simulink library "Lib_EMTAT"  (R2021b)
settings: Solver=VariableStepAuto  StartTime=0.0  StopTime=10.0  RelTol=1e-3
undefined symbols (not defined in the file or in its folder): A_M, B_M, Cj, component_degradation_input, Cs, E0_M, f_sw, K_M, MWS, Q_M, Q_rr, r_c, r_D, R_M, Rj, Ru, SNR_DX_M, SNR_IC_M, SNR_Mn_M, SNR_Mx_M, SOC_Init_M, u_ce0, u_D0
libraries: $bdroot x82, simulink x23, Lib_Dyn_StateSpace_EMTAT x3, PB_Library_Master_Working x1
(part 5 of 7)

== system Lib_EMTAT/Components/Power Flow/Mechanical Shaft ==
  note: Units
      | J : lb-ft-s^2
      | B : lb-ft-s
  T : Inport
  Fail? : Inport  Port=2
  N : Inport  Port=3
  Abs : Abs
  Bus Creator : BusCreator  Inputs=5
  Divide : Product  Inputs=*/
  Failure Determination : Subsystem
  Inertia (slug-ft^2 or lbf-ft-s^2) : Constant  Value=J
  RPM to rad/s : Gain  Gain=(2*pi)/60
  Shaft Break Failure : Subsystem
  Sum : Sum  Inputs=|+-
  "Viscous Damping Coefficient, lbf-ft-s" : Gain  Gain=B
  lbf-ft to Btu : Gain  Gain=0.00128507
  rad/s^2 to RPM/s : Gain  Gain=60/(2*pi)
  Outputs : Outport
  Heat : Outport  Port=2
  Ndot : Outport  Port=3
  wires:
  Shaft Break Failure/1("T ") -> Sum/1
  [SBFail] -> Bus Creator/5  "SBFail"
  RPM to rad/s/1 -> "Viscous Damping Coefficient, lbf-ft-s"/1
  [SBFail] -> Shaft Break Failure/1(Failed?)
  Fail?/1 -> Failure Determination/1(Fail?)
  Failure Determination/1(SBFail) -> [SBFail]
  N/1 -> RPM to rad/s/1, [N]
  [Ndot] -> Bus Creator/3  "Ndot"
  Inertia (slug-ft^2 or lbf-ft-s^2)/1 -> Divide/2
  Bus Creator/1 -> Outputs/1
  rad/s^2 to RPM/s/1 -> [Ndot], Ndot/1
  Divide/1 -> rad/s^2 to RPM/s/1
  [Tnet] -> Bus Creator/1  "Tnet"
  [N] -> Bus Creator/2  "N"
  [Heat] -> Bus Creator/4  "Heat"
  Abs/1 -> Heat/1, [Heat]
  Sum/1 -> [Tnet], Divide/1
  "Viscous Damping Coefficient, lbf-ft-s"/1 -> Sum/2, lbf-ft to Btu/1
  lbf-ft to Btu/1 -> Abs/1
  T/1 -> Shaft Break Failure/2(T)

== system Lib_EMTAT/Components/Power Flow/Power Supply (Set Voltage) ==
  V* : Inport
  Idmd : Inport  Port=2
  Bus Creator : BusCreator  Inputs=3
  Divide : Product  Inputs=**
  MATLAB Function : MATLAB Function  TreatAsAtomicUnit=on
  Outputs : Outport
  Vout : Outport  Port=2
  wires:
  [Pdmd] -> Bus Creator/3  "Pdmd"
  [Idmdsum] -> Bus Creator/2  "Idmdsum"
  [Vout] -> Bus Creator/1  "Vout"
  Divide/1 -> [Pdmd]
  Bus Creator/1 -> Outputs/1
  V*/1 -> Vout/1, Divide/1, [Vout]
  MATLAB Function/1(y) -> [Idmdsum], Divide/2  "Idmdsum"
  Idmd/1 -> MATLAB Function/1(u)

== system Lib_EMTAT/Components/Power Flow/Resistive Load Bank ==
  V : Inport
  "P* " : Inport  Port=2
  Fail? : Inport  Port=3
  Abs1 : Abs
  Bus Creator : BusCreator  Inputs=5
  Divide2 : Product  Inputs=**
  Failure Determination : Subsystem
  Fix Divide By Zero. : Subsystem
  Fix Divide By Zero.1 : Subsystem
  Open Circuit Failure - Line to Neutral Voltage : Subsystem
  Square : Math  Operator=square  SaturateOnIntegerOverflow=on
  Outputs : Outport
  Ploss : Outport  Port=2
  Iin : Outport  Port=3
  wires:
  Fix Divide By Zero.1/1(I) -> Open Circuit Failure - Line to Neutral Voltage/2(I)
  [OCFail] -> Open Circuit Failure - Line to Neutral Voltage/1(Failed?)
  Fail?/1 -> Failure Determination/1(Fail?)
  Failure Determination/1(OCFail) -> [OCFail]
  Abs1/1 -> Fix Divide By Zero./2(abs(Pset))
  Fix Divide By Zero./1(R) -> [R], Divide2/2
  Bus Creator/1 -> Outputs/1
  Square/1 -> Divide2/1, Fix Divide By Zero./1(I^2)
  "P* "/1 -> [Pset], Abs1/1, Fix Divide By Zero.1/2(Pset)  "Pset"
  V/1 -> [V], Fix Divide By Zero.1/1(V)  "V"
  Divide2/1 -> [Ploss], Ploss/1
  [V] -> Bus Creator/1  "V"
  [I] -> Bus Creator/2  "I"
  [Pset] -> Bus Creator/3  "Pset"
  [R] -> Bus Creator/4  "R"
  [Ploss] -> Bus Creator/5  "Ploss"
  Open Circuit Failure - Line to Neutral Voltage/1("I ") -> Square/1, [I], Iin/1

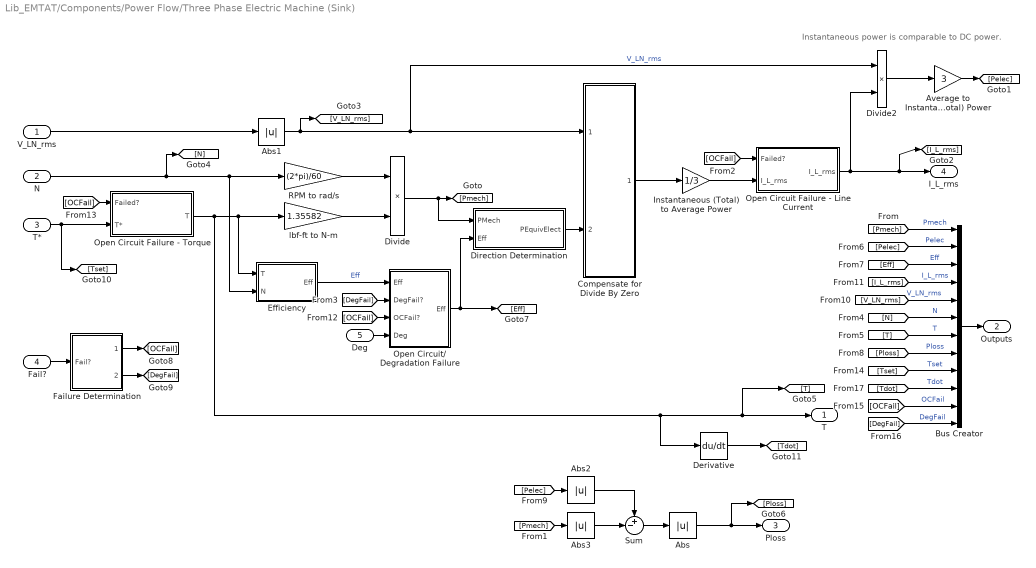
== system Lib_EMTAT/Components/Power Flow/Three Phase Electric Machine (Sink) ==
  note: Instantaneous power is comparable to DC power.
  V_LN_rms : Inport
  N : Inport  Port=2
  T* : Inport  Port=3
  Fail? : Inport  Port=4
  Deg : Inport  Port=5
  Abs{,1..3} (4 alike) : Abs
  Average to Instantaneous (Total) Power : Gain  Gain=3
  Bus Creator : BusCreator  Inputs=12
  Compensate for Divide By Zero : Subsystem
  Derivative : Derivative
  Direction Determination : Subsystem
  Divide : Product  Inputs=**
  Divide2 : Product  Inputs=**
  Efficiency : Subsystem
  Failure Determination : Subsystem
  Instantaneous (Total) to Average Power : Gain  Gain=1/3
  Open Circuit Failure - Line Current : Subsystem
  Open Circuit Failure - Torque : Subsystem
  Open Circuit/ Degradation Failure : Subsystem
  RPM to rad/s : Gain  Gain=(2*pi)/60
  Sum : Sum  Inputs=+-|
  lbf-ft to N-m : Gain  Gain=1.35582
  T : Outport
  Outputs : Outport  Port=2
  Ploss : Outport  Port=3
  I_L_rms : Outport  Port=4
  wires:
  [Tdot] -> Bus Creator/10  "Tdot"
  Derivative/1 -> [Tdot]
  [DegFail] -> Bus Creator/12  "DegFail"
  [OCFail] -> Bus Creator/11  "OCFail"
  [Tset] -> Bus Creator/9  "Tset"
  T*/1 -> [Tset], Open Circuit Failure - Torque/2(T*)
  [OCFail] -> Open Circuit Failure - Torque/1(Failed?)
  [OCFail] -> Open Circuit/ Degradation Failure/3(OCFail?)
  Fail?/1 -> Failure Determination/1(Fail?)
  Deg/1 -> Open Circuit/ Degradation Failure/4(Deg)
  [DegFail] -> Open Circuit/ Degradation Failure/2(DegFail?)
  Open Circuit/ Degradation Failure/1("Eff ") -> [Eff], Direction Determination/2(Eff)
  Failure Determination/2(DegFail) -> [DegFail]
  Failure Determination/1(OCFail) -> [OCFail]
  [OCFail] -> Open Circuit Failure - Line Current/1(Failed?)
  Instantaneous (Total) to Average Power/1 -> Open Circuit Failure - Line Current/2(I_L_rms)
  Open Circuit Failure - Line Current/1("I_L_rms ") -> I_L_rms/1, [I_L_rms], Divide2/2
  Compensate for Divide By Zero/1(I_L_rms) -> Instantaneous (Total) to Average Power/1
  [N] -> Bus Creator/6  "N"
  [I_L_rms] -> Bus Creator/4  "I_L_rms"
  [V_LN_rms] -> Bus Creator/5  "V_LN_rms"
  Abs1/1 -> [V_LN_rms], Divide2/1, Compensate for Divide By Zero/1(V_LN_rms)  "V_LN_rms"
  Abs3/1 -> Sum/2
  [Pmech] -> Abs3/1
  Abs2/1 -> Sum/1
  [Pelec] -> Abs2/1
  Bus Creator/1 -> Outputs/1
  Efficiency/1(Eff) -> Open Circuit/ Degradation Failure/1(Eff)  "Eff"
  V_LN_rms/1 -> Abs1/1
  lbf-ft to N-m/1 -> Divide/2
  RPM to rad/s/1 -> Divide/1
  Open Circuit Failure - Torque/1("T  ") -> Efficiency/1(T), lbf-ft to N-m/1, T/1, [T], Derivative/1
  Divide/1 -> [Pmech], Direction Determination/1(PMech)
  [Pmech] -> Bus Creator/1  "Pmech"
  Divide2/1 -> Average to Instantaneous (Total) Power/1
  [T] -> Bus Creator/7  "T"
  [Eff] -> Bus Creator/3  "Eff"
  [Ploss] -> Bus Creator/8  "Ploss"
  Sum/1 -> Abs/1
  [Pelec] -> Bus Creator/2  "Pelec"
  Abs/1 -> [Ploss], Ploss/1
  Direction Determination/1(PEquivElect) -> Compensate for Divide By Zero/2(PEquivElect)
  N/1 -> Efficiency/2(N), RPM to rad/s/1, [N]
  Average to Instantaneous (Total) Power/1 -> [Pelec]

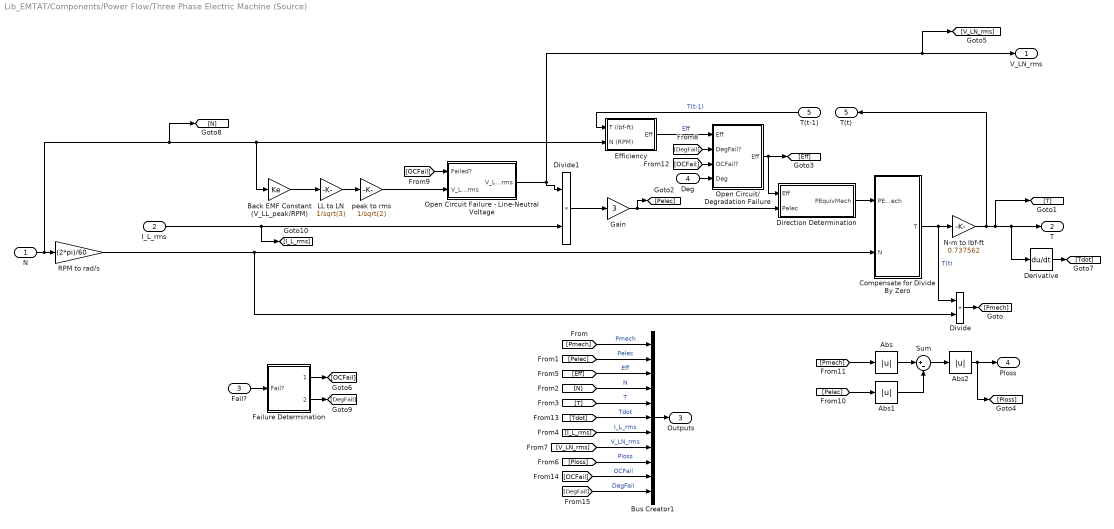
== system Lib_EMTAT/Components/Power Flow/Three Phase Electric Machine (Source) ==
  N : Inport
  I_L_rms : Inport  Port=2
  Fail? : Inport  Port=3
  Deg : Inport  Port=4
  T(t-1) : Inport  Port=5
  Abs : Abs
  Abs1 : Abs
  Abs2 : Abs
  Back EMF Constant (V_LL_peak/RPM) : Gain  Gain=Ke
  Bus Creator1 : BusCreator  Inputs=11
  Compensate for Divide By Zero : Subsystem
  Derivative : Derivative
  Direction Determination : Subsystem
  Divide : Product  Inputs=**
  Divide1 : Product  Inputs=**
  Efficiency : Subsystem
  Failure Determination : Subsystem
  Gain : Gain  Gain=3
  LL to LN : Gain  Gain=1/sqrt(3)
  N-m to lbf-ft : Gain  Gain=0.737562
  Open Circuit Failure - Line-Neutral Voltage : Subsystem
  Open Circuit/ Degradation Failure : Subsystem
  RPM to rad/s : Gain  Gain=(2*pi)/60
  Sum : Sum  Inputs=|+-
  peak to rms : Gain  Gain=1/sqrt(2)
  V_LN_rms : Outport
  T : Outport  Port=2
  Outputs : Outport  Port=3
  Ploss : Outport  Port=4
  T(t) : Outport  Port=5
  wires:
  [DegFail] -> Bus Creator1/11  "DegFail"
  [OCFail] -> Bus Creator1/10  "OCFail"
  [Tdot] -> Bus Creator1/6  "Tdot"
  Derivative/1 -> [Tdot]
  peak to rms/1 -> Open Circuit Failure - Line-Neutral Voltage/2(V_LN_rms)
  Open Circuit Failure - Line-Neutral Voltage/1("V_LN_rms ") -> V_LN_rms/1, [V_LN_rms], Divide1/1
  [OCFail] -> Open Circuit Failure - Line-Neutral Voltage/1(Failed?)
  Open Circuit/ Degradation Failure/1("Eff ") -> Direction Determination/1(Eff), [Eff]
  Deg/1 -> Open Circuit/ Degradation Failure/4(Deg)
  [DegFail] -> Open Circuit/ Degradation Failure/2(DegFail?)
  Efficiency/1(Eff) -> Open Circuit/ Degradation Failure/1(Eff)  "Eff"
  [OCFail] -> Open Circuit/ Degradation Failure/3(OCFail?)
  Failure Determination/1(OCFail) -> [OCFail]
  Failure Determination/2(DegFail) -> [DegFail]
  Fail?/1 -> Failure Determination/1(Fail?)
  N-m to lbf-ft/1 -> T/1, Derivative/1, [T], T(t)/1
  Gain/1 -> Direction Determination/2(Pelec), [Pelec]
  LL to LN/1 -> peak to rms/1
  [Pmech] -> Abs/1
  [Pelec] -> Abs1/1
  Divide/1 -> [Pmech]
  Abs2/1 -> Ploss/1, [Ploss]
  Sum/1 -> Abs2/1
  Abs1/1 -> Sum/2
  Abs/1 -> Sum/1
  Bus Creator1/1 -> Outputs/1
  Direction Determination/1(PEquivMech) -> Compensate for Divide By Zero/1(PEquivMech)
  T(t-1)/1 -> Efficiency/1(T (lbf-ft))  "T(t-1)"
  Compensate for Divide By Zero/1(T) -> N-m to lbf-ft/1, Divide/1  "T(t)"
  Divide1/1 -> Gain/1
  Back EMF Constant (V_LL_peak/RPM)/1 -> LL to LN/1
  N/1 -> RPM to rad/s/1, Efficiency/2(N (RPM)), Back EMF Constant (V_LL_peak/RPM)/1, [N]
  [V_LN_rms] -> Bus Creator1/8  "V_LN_rms"
  [I_L_rms] -> Bus Creator1/7  "I_L_rms"
  [Eff] -> Bus Creator1/3  "Eff"
  [T] -> Bus Creator1/5  "T"
  [N] -> Bus Creator1/4  "N"
  [Pmech] -> Bus Creator1/1  "Pmech"
  [Ploss] -> Bus Creator1/9  "Ploss"
  [Pelec] -> Bus Creator1/2  "Pelec"
  RPM to rad/s/1 -> Divide/2, Compensate for Divide By Zero/2(N)
  I_L_rms/1 -> Divide1/2, [I_L_rms]

== system Lib_EMTAT/Numerical Methods/Jacobian Calculator/Counter ==
  Reset : Inport
  Constant : Constant
  Constant1 : Constant  Value=N_Ind_M
  Constant2 : Constant  Value=3
  Logical Operator1 : Logic  Operator=NOT  AllPortsSameDT=off  OutDataTypeStr=boolean
  MinMax1 : MinMax  Inputs=2
  Product : Product  RndMeth=Zero
  Relational Operator : RelationalOperator  Operator=>  OutDataTypeStr=boolean  RndMeth=Nearest
  Sum : Sum  Inputs=|++
  Sum1 : Sum  Inputs=|++
  Unit Delay : UnitDelay  SampleTime=-1  HasFrameUpgradeWarning=on
  Enable : Outport
  Iteration : Outport  Port=2
  wires:
  Constant/1 -> Sum/1
  Product/1 -> MinMax1/1
  Sum/1 -> MinMax1/2
  Unit Delay/1 -> Sum/2
  MinMax1/1 -> Unit Delay/1, Iteration/1, Relational Operator/2
  Relational Operator/1 -> Enable/1
  Logical Operator1/1 -> Product/2
  Reset/1 -> Logical Operator1/1
  Sum1/1 -> Relational Operator/1, Product/1
  Constant2/1 -> Sum1/2
  Constant1/1 -> Sum1/1

== system Lib_EMTAT/Numerical Methods/Jacobian Calculator/Jacobian ==
  Iteration : Inport
  Per : Inport  Port=2
  f(x_p) : Inport  Port=3
  Xo : Inport  Port=4
  Enable : EnablePort
  Jacobian Calc : MATLAB Function  TreatAsAtomicUnit=on
  Unit Delay : UnitDelay  InitialCondition=zeros(size(N_Per_M,2),size(N_Per_M,2))  SampleTime=-1  HasFrameUpgradeWarning=on
  Unit Delay1 : UnitDelay  InitialCondition=zeros(size(N_Per_M,2),prod(size(N_Per_M))+1)  SampleTime=-1  HasFrameUpgradeWarning=on
  Unit Delay2 : UnitDelay  InitialCondition=zeros(size(N_Per_M,2),1)  SampleTime=-1  HasFrameUpgradeWarning=on
  Unit Delay3 : UnitDelay  SampleTime=-1  HasFrameUpgradeWarning=on
  x_p : Outport
  Inv(J) : Outport  Port=2
  J : Outport  Port=3
  y_State : Outport  Port=4
  JacFailed : Outport  Port=5
  wires:
  Jacobian Calc/1(XpOut) -> x_p/1
  Xo/1 -> Jacobian Calc/4(XoIn)
  Per/1 -> Jacobian Calc/3(PerIn)
  Iteration/1 -> Jacobian Calc/1(IterationIn)
  Jacobian Calc/3(JOut) -> Unit Delay/1, J/1
  Jacobian Calc/2(InvJOut) -> Inv(J)/1
  Unit Delay/1 -> Jacobian Calc/5(JStateIn)
  Jacobian Calc/4(y_StateOut) -> Unit Delay1/1, y_State/1
  Unit Delay1/1 -> Jacobian Calc/6(y_StateIn)
  f(x_p)/1 -> Unit Delay2/1
  Unit Delay2/1 -> Jacobian Calc/2(y_xpIn)
  Jacobian Calc/5(ErSv) -> Unit Delay3/1, JacFailed/1
  Unit Delay3/1 -> Jacobian Calc/7(Er)

== system Lib_EMTAT/Numerical Methods/Newton Raphson Solver/NR Update ==
  f(x) : Inport
  inv(J) : Inport  Port=2
  x(n) : Inport  Port=3
  Enable : EnablePort
  Bounding : Subsystem
  MatrixMult : Subsystem
  Sum : Sum  Inputs=|-+
  dxLimit1 : Subsystem
  x(n+1) : Outport
  wires:
  x(n)/1 -> Sum/2
  Bounding/1(x(n+1)Lim) -> x(n+1)/1
  inv(J)/1 -> MatrixMult/2(inv(f'(x(n))))
  MatrixMult/1(DTS) -> dxLimit1/1(dx)
  Sum/1 -> Bounding/1(x(n+1)raw)
  f(x)/1 -> MatrixMult/1(f(x(n))), dxLimit1/2(f(x(n)))
  dxLimit1/1(dx_limited) -> Sum/1

== system Lib_EMTAT/Solvers/Iterative NR Solver w JacobianCalc/JC w Reset ==
  note: Reset Jacobian Calculator after SJacobianAttempts_M
  f(x) : Inport  PortDimensions=length(SNR_IC_M)
  Iter : Inport  Port=2  PortDimensions=1
  x(n+1) : Inport  Port=3
  Enable : EnablePort
  Constant : Constant  Value=SNR_IC_M
  Constant1 : Constant  Value=SJacobianAttempts_M  OutDataTypeStr=uint32
  Jacobian Calculator : $bdroot/Numerical Methods/Jacobian Calculator  N_Per_M=SJac_Per_M
  Product : Product  RndMeth=Zero
  Relational Operator : RelationalOperator  Operator===  OutDataTypeStr=boolean  RndMeth=Nearest
  Switch : Switch  Criteria=u2 ~= 0  Threshold=1
  Terminator3 : Terminator
  Unit Delay : UnitDelay  InitialCondition=ones(length(SNR_IC_M),1)  SampleTime=-1  HasFrameUpgradeWarning=on
  J : Outport  PortDimensions=[length(SNR_IC_M),length(SNR_IC_M)]
  JacFailed : Outport  Port=2  PortDimensions=1
  X_out : Outport  Port=3  PortDimensions=length(SNR_IC_M)
  JC_Active : Outport  Port=4  PortDimensions=1
  inv(J) : Outport  Port=5  PortDimensions=[length(SNR_IC_M),length(SNR_IC_M)]
  wires:
  f(x)/1 -> Jacobian Calculator/2
  Jacobian Calculator/5 -> inv(J)/1
  Unit Delay/1 -> Switch/3, Jacobian Calculator/3
  x(n+1)/1 -> Unit Delay/1
  Jacobian Calculator/1 -> J/1  "J"
  Constant/1 -> Product/2
  Relational Operator/1 -> Jacobian Calculator/1
  Product/1 -> X_out/1
  Jacobian Calculator/2 -> Switch/1
  Switch/1 -> Product/1
  Jacobian Calculator/4 -> Switch/2, JC_Active/1
  Constant1/1 -> Relational Operator/2
  Iter/1 -> Relational Operator/1
  Jacobian Calculator/3 -> Terminator3/1
  Jacobian Calculator/6 -> JacFailed/1  "JacFalied"

== system Lib_EMTAT/Solvers/Iterative NR Solver w JacobianCalc/NRwCond ==
  note: Enable NR when conditions are not met
      | and Jacobian Calculator is not active
  f(x) : Inport  PortDimensions=length(SNR_IC_M)
  JC_Active : Inport  Port=2  PortDimensions=1
  inv(f'(x)) : Inport  Port=3  PortDimensions=[length(SNR_IC_M),length(SNR_IC_M)]
  Enable : EnablePort
  Iteration Conditions : Subsystem
  Logical Operator : Logic  Operator=NOT  AllPortsSameDT=off  OutDataTypeStr=boolean
  Logical Operator1 : Logic  AllPortsSameDT=off  OutDataTypeStr=boolean
  Newton Raphson Solver : $bdroot/Numerical Methods/Newton Raphson Solver  NR_IC_M=SNR_IC_M./abs(SNR_IC_M)  NR_dx_Lim_M=SNR_DX_M  NR_Mx_Lim_M=SNR_Mx_M./abs(SNR_IC_M)  NR_Mn_Lim_M=SNR_Mn_M./abs(SNR_IC_M)  BlkNm_M=double(gcb)
  Terminator : Terminator
  CCnd : Outport  PortDimensions=1
  x(n+1) : Outport  Port=2  PortDimensions=length(SNR_IC_M)
  wires:
  f(x)/1 -> Newton Raphson Solver/3, Iteration Conditions/1(f(x))
  JC_Active/1 -> Logical Operator/1
  Newton Raphson Solver/2 -> x(n+1)/1
  Newton Raphson Solver/1 -> Terminator/1
  inv(f'(x))/1 -> Newton Raphson Solver/2
  Logical Operator1/1 -> Newton Raphson Solver/1
  Logical Operator/1 -> Logical Operator1/1
  Iteration Conditions/1(Condition) -> Logical Operator1/2, CCnd/1

== system Lib_EMTAT/Solvers/SS NR Solver w JacobianCalc /JacCalc w Reset ==
  f(x) : Inport  PortDimensions=length(SNR_IC_M)
  CCnd : Inport  Port=2  PortDimensions=1
  x(n+1) : Inport  Port=3  PortDimensions=length(SNR_IC_M)
  Enable : EnablePort
  Constant : Constant  Value=SNR_IC_M
  JC_Reset counter : Subsystem
  Jacobian Calculator1 : $bdroot/Numerical Methods/Jacobian Calculator  N_Per_M=SJac_Per_M
  Product : Product  RndMeth=Zero
  Switch : Switch  Criteria=u2 ~= 0  Threshold=1
  Terminator3 : Terminator
  Unit Delay2 : UnitDelay  InitialCondition=ones(length(SNR_IC_M),1)  SampleTime=-1  HasFrameUpgradeWarning=on
  X_out : Outport  PortDimensions=length(SNR_IC_M)
  JC_Active : Outport  Port=2  PortDimensions=1
  inv(J) : Outport  Port=3  PortDimensions=[length(SNR_IC_M),length(SNR_IC_M)]
  J : Outport  Port=4  PortDimensions=[length(SNR_IC_M),length(SNR_IC_M)]
  JacFailed : Outport  Port=5  PortDimensions=1
  wires:
  Jacobian Calculator1/3 -> Terminator3/1
  Jacobian Calculator1/2 -> Switch/1
  Jacobian Calculator1/4 -> JC_Active/1, [JC_Active]
  Unit Delay2/1 -> Switch/3, Jacobian Calculator1/3
  Constant/1 -> Product/2
  Jacobian Calculator1/5 -> inv(J)/1
  [JC_Active] -> JC_Reset counter/1(Reset Counter)
  Switch/1 -> Product/1
  Jacobian Calculator1/1 -> J/1  "J"
  Product/1 -> X_out/1
  JC_Reset counter/1(JC_Reset) -> Jacobian Calculator1/1
  x(n+1)/1 -> Unit Delay2/1
  CCnd/1 -> JC_Reset counter/2(Count Condition)
  [JC_Active] -> Switch/2
  f(x)/1 -> Jacobian Calculator1/2
  Jacobian Calculator1/6 -> JacFailed/1

== system Lib_EMTAT/Solvers/SS NR Solver w JacobianCalc /NewRaph w Cond ==
  f(x(n)) : Inport  PortDimensions=length(SNR_IC_M)
  JC_Active : Inport  Port=2  PortDimensions=1
  inv(f'x(n)) : Inport  Port=3  PortDimensions=[length(SNR_IC_M),length(SNR_IC_M)]
  Enable : EnablePort
  Logical Operator : Logic  Operator=NOT  AllPortsSameDT=off  OutDataTypeStr=boolean
  Logical Operator1 : Logic  AllPortsSameDT=off  OutDataTypeStr=boolean
  Logical Operator2 : Logic  Operator=NOT  AllPortsSameDT=off  OutDataTypeStr=boolean
  Newton Raphson Solver : $bdroot/Numerical Methods/Newton Raphson Solver  NR_IC_M=SNR_IC_M./abs(SNR_IC_M)  NR_dx_Lim_M=SNR_DX_M  NR_Mx_Lim_M=SNR_Mx_M./abs(SNR_IC_M)  NR_Mn_Lim_M=SNR_Mn_M./abs(SNR_IC_M)  BlkNm_M=double(gcb)
  Terminator : Terminator
  conditions : Subsystem
  Converged : Outport  PortDimensions={1,[length(SNR_IC_M),length(SNR_IC_M)]}
  CCnd : Outport  Port=2  PortDimensions=1
  x(n+1) : Outport  Port=3  PortDimensions=length(SNR_IC_M)
  wires:
  Logical Operator/1 -> Logical Operator1/1
  Logical Operator1/1 -> Newton Raphson Solver/1
  conditions/1(Condition) -> Logical Operator2/1, CCnd/1, Logical Operator1/2
  Logical Operator2/1 -> Converged/1  "Converged"
  JC_Active/1 -> Logical Operator/1
  inv(f'x(n))/1 -> Newton Raphson Solver/2
  Newton Raphson Solver/1 -> Terminator/1
  Newton Raphson Solver/2 -> x(n+1)/1
  f(x(n))/1 -> Newton Raphson Solver/3, conditions/1(f(x))

== system Lib_EMTAT/Components/Physics-Based/Boost Converter/DC - DC Converter ==
  note: the aDF must decrease L_M
  note: Power B
  note: Current B
  note: Power B
  VIn : Inport
  x : Inport  Port=2
  d : Inport  Port=3
  dt : Inport  Port=4
  I_Demand : Inport  Port=5
  P loss : Inport  Port=6
  "T_Ambient " : Inport  Port=7
  " Dynamic State" : Subsystem  TreatAsAtomicUnit=on
  "1=dynamic, 0=static" : Display
  Add : Sum
  Bus Creator1 : BusCreator  Inputs=3
  Bus Creator3 : BusCreator  Inputs=3
  Bus Selector : BusSelector  OutputSignals=x,xdot,VB
  Constant : Constant  Value=[0, 1/C_M; -1/L_M, -(Ron_M+RC_M+RL_M)/L_M]  VectorParams1D=off
  Display : Display
  Divide : Product  Inputs=*/
  If : If
  MATLAB Function : MATLAB Function  TreatAsAtomicUnit=on
  Mux : Mux  Inputs=2
  Product3 : Product
  Steady State : Subsystem  TreatAsAtomicUnit=on
  Switch : Switch  Criteria=u2 ~= 0
  xdot : Constant  Value=zeros(2,1)  VectorParams1D=off
  VOut : Outport  VectorParamsAs1DForOutWhenUnconnected=off
  x_dot : Outport  Port=2  VectorParamsAs1DForOutWhenUnconnected=off
  x_new : Outport  Port=3  VectorParamsAs1DForOutWhenUnconnected=off
  I_Demanded : Outport  Port=4  VectorParamsAs1DForOutWhenUnconnected=off
  switchDyn : Outport  Port=5  VectorParamsAs1DForOutWhenUnconnected=off
  wires:
  "T_Ambient "/1 -> Steady State/3("T_Ambient "), Display/1
  Add/1 -> [PwrA]
  Mux/1 -> " Dynamic State"/2(u), Steady State/1(u)
  I_Demand/1 -> [IB], Mux/2
  [VA] -> Mux/1
  [x] -> x_new/1
  Bus Creator3/1 -> Switch/1
  Bus Selector/1 -> [x]  "<x>"
  Bus Selector/2 -> [xdot]  "<xdot>"
  Bus Selector/3 -> [VB]  "<VB>"
  xdot/1 -> Bus Creator1/2  "xdot"
  Steady State/2(VB) -> Bus Creator1/3  "VB"
  " Dynamic State"/1(xdot) -> Bus Creator3/2  "xdot"
  " Dynamic State"/2(VB) -> Bus Creator3/3  "VB"
  Switch/1 -> Bus Selector/1
  P loss/1 -> Add/2
  [PwrB] -> Add/1
  [xdot] -> x_dot/1
  d/1 -> " Dynamic State"/3(d), Steady State/2(d)
  x/1 -> " Dynamic State"/1(x), Bus Creator3/1  "x"
  Steady State/1(x) -> Bus Creator1/1  "x"
  dt/1 -> MATLAB Function/2(dt)
  If/2 -> Steady State/Action
  Constant/1 -> MATLAB Function/1(A1)
  If/1 -> " Dynamic State"/Action
  MATLAB Function/1(y) -> If/1, switchDyn/1, Switch/2, "1=dynamic, 0=static"/1
  [IA] -> I_Demanded/1
  [VA] -> Divide/2
  Divide/1 -> [IA]
  [PwrA] -> Divide/1
  [IB] -> Product3/2
  VIn/1 -> [VA]
  [VB] -> VOut/1  "V"
  Product3/1 -> [PwrB]
  [VB] -> Product3/1
  Bus Creator1/1 -> Switch/3

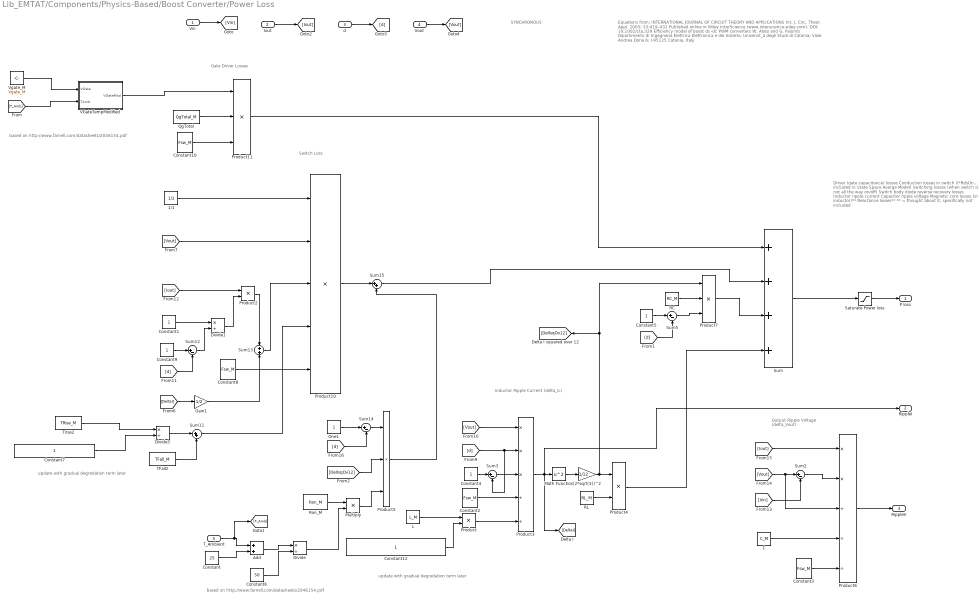
== system Lib_EMTAT/Components/Physics-Based/Boost Converter/Power Loss  ==
  note: Gate Driver Losses
  note: Output Ripple Voltage
      | (delta_Vout)
  note: Inductor Ripple Current
      | (delta_iL)
  note: Driver (gate capacitance) losses
      | Conduction losses in switch (I*RdsOn... included in State Space Averge Model)
      | Switching losses (when switch is not all the way on/off)
      | Switch body diode reverse recovery losses
      | Inductor ripple current
      | Capacitor ripple voltage
      | Magnetic core losses (in inductor)**
      | Reactance losses**
      | ** = thought about it, specifically not included
  note: SYNCHRONOUS
  note: Switch Loss
  note: Equations from:
      | INTERNATIONAL JOURNAL OF CIRCUIT THEORY AND APPLICATIONS
      | Int. J. Circ. Theor. Appl. 2005; 33:419–432
      | Published online in Wiley InterScience (www.interscience.wiley.com). DOI: 10.1002/cta.329
      | Efficiency model of boost dc–dc PWM converters
      | W. Aloisi and G. Palumb
      | Dipartimento di Ingegneria Elettrica Elettronica e dei Sistemi; Universit_a degli Studi di Catania;
      | Viale Andrea Doria 6; I-95125 Catania, Italy
  note: based on http://www.farnell.com/datasheets/2046154.pdf
  note: based on http://www.farnell.com/datasheets/2046154.pdf
  note: update with gradual degredation term later
  note: update with gradual degredation term later
  Vin : Inport
  Iout : Inport  Port=2
  d : Inport  Port=3
  Vout : Inport  Port=4
  "T_Ambient " : Inport  Port=5
  (2*sqrt(3))^2 : Gain  Gain=1/12
  1/1 : Constant  Value=1/2  VectorParams1D=off
  Add : Sum
  C : Constant  Value=C_M  VectorParams1D=off
  Constant : Constant  Value=25
  Constant{1,4..5,7,9,12} (6 alike) : Constant
  Constant{2..3,8,10} (4 alike) : Constant  Value=Fsw_M
  Constant6 : Constant  Value=50
  Divide : Product  Inputs=*/
  Divide1 : Product  Inputs=*/
  Divide3 : Product  Inputs=*/
  Gain1 : Gain  Gain=1/2
  L : Constant  Value=L_M  VectorParams1D=off
  Math Function : Math  Operator=square  SignedPower=on  SaturateOnIntegerOverflow=on
  Multiply : Product
  One1 : Constant  VectorParams1D=off
  Product : Product
  Product10 : Product  Inputs=5
  Product11 : Product  Inputs=3
  Product2 : Product
  Product3 : Product  Inputs=***//
  Product4 : Product
  Product5 : Product  Inputs=3
  Product6 : Product  Inputs=**///
  Product7 : Product  Inputs=3
  QgTotal : Constant  Value=QgTotal_M  VectorParams1D=off
  RC : Constant  Value=RC_M  VectorParams1D=off
  RL : Constant  Value=RL_M  VectorParams1D=off
  Ron_M : Constant  Value=Ron_M
  Saturate Power loss : Saturate  UpperLimit=inf  LowerLimit=0
  Sum : Sum  Inputs=++++
  Sum11 : Sum  Inputs=|++
  Sum{2..3,5,12,14} (5 alike) : Sum  Inputs=|+-
  Sum13 : Sum
  Sum15 : Sum  Inputs=|++
  TFall2 : Constant  Value=TFall_M  VectorParams1D=off
  Trise2 : Constant  Value=TRise_M  VectorParams1D=off
  VGateTempModified : Subsystem
  "Vgate_M " : Constant  Value=Vgate_M
  " P loss" : Outport  VectorParamsAs1DForOutWhenUnconnected=off
  RippleI : Outport  Port=2  VectorParamsAs1DForOutWhenUnconnected=off
  RippleV : Outport  Port=3  VectorParamsAs1DForOutWhenUnconnected=off
  wires:
  VGateTempModified/1(VGateMod) -> Product11/1
  [T_Amb] -> VGateTempModified/2(TAmb)
  "Vgate_M "/1 -> VGateTempModified/1(VGate)
  Multiply/1 -> Product5/3
  Divide/1 -> Multiply/2
  Add/1 -> Divide/1
  Constant6/1 -> Divide/2
  Constant/1 -> Add/2
  "T_Ambient "/1 -> Add/1, [T_Amb]
  Sum15/1 -> Sum/2
  Product11/1 -> Sum/1
  Product7/1 -> Sum/3
  Product4/1 -> Sum/4
  QgTotal/1 -> Product11/2
  Product5/1 -> Sum15/2
  Product10/1 -> Sum15/1
  [DelIsqOv12] -> Product5/2
  Sum14/1 -> Product5/1
  One1/1 -> Sum14/1
  [d] -> Sum14/2
  Product6/1 -> RippleV/1
  C/1 -> Product6/4
  Sum2/1 -> Product6/2
  [Vin] -> Sum2/2
  [Vout] -> Sum2/1, Product6/3
  [Iout] -> Product6/1
  1/1/1 -> Product10/1
  [Vout] -> Product10/2
  Product2/1 -> Sum13/1
  Sum11/1 -> Product10/4
  Constant1/1 -> Divide1/1
  Divide1/1 -> Product2/2
  Sum12/1 -> Divide1/2
  Sum13/1 -> Product10/3
  Gain1/1 -> Sum13/2
  Constant9/1 -> Sum12/1
  [d] -> Sum12/2
  [DeltaI] -> Gain1/1
  [Iout] -> Product2/1
  Sum5/1 -> Product7/3
  [d] -> Sum5/2
  Constant5/1 -> Sum5/1
  Sum3/1 -> Product3/3
  Constant4/1 -> Sum3/1
  [Vout] -> Product3/1
  Vout/1 -> [Vout]
  [d] -> Product3/2, Sum3/2
  d/1 -> [d]
  Iout/1 -> [Iout]
  Vin/1 -> [Vin]
  Sum/1 -> Saturate Power loss/1
  Saturate Power loss/1 -> " P loss"/1
  RL/1 -> Product4/2
  Product3/1 -> RippleI/1, Math Function/1, [DeltaI]
  (2*sqrt(3))^2/1 -> [DelIsqOv12], Product7/1, Product4/1
  Math Function/1 -> (2*sqrt(3))^2/1
  RC/1 -> Product7/2
  Ron_M/1 -> Multiply/1
  Divide3/1 -> Sum11/1
  Trise2/1 -> Divide3/1
  Constant7/1 -> Divide3/2
  Constant10/1 -> Product11/3
  Constant8/1 -> Product10/5
  Constant2/1 -> Product3/4
  Constant3/1 -> Product6/5
  TFall2/1 -> Sum11/2
  Product/1 -> Product3/5
  L/1 -> Product/1
  Constant12/1 -> Product/2

== system Lib_EMTAT/Components/Physics-Based/Buck Converter/DC - DC Converter ==
  note: Power A
  note: Current A
  note: Power B
  VIn : Inport
  x : Inport  Port=2
  d : Inport  Port=3
  dt : Inport  Port=4
  I_Demand : Inport  Port=5
  P loss : Inport  Port=6
  "T_Ambient " : Inport  Port=7
  " Dynamic State" : Subsystem  TreatAsAtomicUnit=on
  "1=dynamic, 0=static" : Display
  Add : Sum
  Bus Creator1 : BusCreator  Inputs=3
  Bus Creator3 : BusCreator  Inputs=3
  Bus Selector : BusSelector  OutputSignals=x,xdot,VB
  Constant : Constant  Value=[0, 1/C_M; -1/L_M, -(Ron_M+RC_M+RL_M)/L_M]  VectorParams1D=off
  Divide : Product  Inputs=*/
  If : If
  MATLAB Function : MATLAB Function  TreatAsAtomicUnit=on
  Mux : Mux  Inputs=2
  Product3 : Product
  Steady State : Subsystem  TreatAsAtomicUnit=on
  Switch : Switch  Criteria=u2 ~= 0
  xdot : Constant  Value=zeros(2,1)  VectorParams1D=off
  Vout : Outport  VectorParamsAs1DForOutWhenUnconnected=off
  x_dot : Outport  Port=2  VectorParamsAs1DForOutWhenUnconnected=off
  x_new : Outport  Port=3  VectorParamsAs1DForOutWhenUnconnected=off
  I_Demanded : Outport  Port=4  VectorParamsAs1DForOutWhenUnconnected=off
  switchDyn : Outport  Port=5  VectorParamsAs1DForOutWhenUnconnected=off
  wires:
  Bus Creator1/1 -> Switch/3
  [VB] -> Vout/1  "V"
  VIn/1 -> [VA]
  [IB] -> Product3/2
  [IA] -> I_Demanded/1
  MATLAB Function/1(y) -> "1=dynamic, 0=static"/1, Switch/2, switchDyn/1, If/1
  If/1 -> " Dynamic State"/Action
  Constant/1 -> MATLAB Function/1(A1)
  If/2 -> Steady State/Action
  dt/1 -> MATLAB Function/2(dt)
  Steady State/1(x) -> Bus Creator1/1  "x"
  x/1 -> Bus Creator3/1, " Dynamic State"/1(x)  "x"
  d/1 -> Steady State/2(d), " Dynamic State"/3(d)
  [xdot] -> x_dot/1
  P loss/1 -> Add/2
  Switch/1 -> Bus Selector/1
  " Dynamic State"/2(VB) -> Bus Creator3/3  "VB"
  " Dynamic State"/1(xdot) -> Bus Creator3/2  "xdot"
  Steady State/2(VB) -> Bus Creator1/3  "VB"
  xdot/1 -> Bus Creator1/2  "xdot"
  Bus Selector/3 -> [VB]  "<VB>"
  Bus Selector/2 -> [xdot]  "<xdot>"
  Bus Selector/1 -> [x]  "<x>"
  Bus Creator3/1 -> Switch/1
  [x] -> x_new/1
  [VA] -> Mux/1
  Mux/1 -> Steady State/1(u), " Dynamic State"/2(u)
  "T_Ambient "/1 -> Steady State/3("T_Ambient ")
  I_Demand/1 -> [IB], Mux/2
  [VB] -> Product3/1  "V"
  Product3/1 -> [PwrB]
  Divide/1 -> [IA]
  [PwrB] -> Add/1
  Add/1 -> [PwrA]
  [PwrA] -> Divide/1
  [VA] -> Divide/2

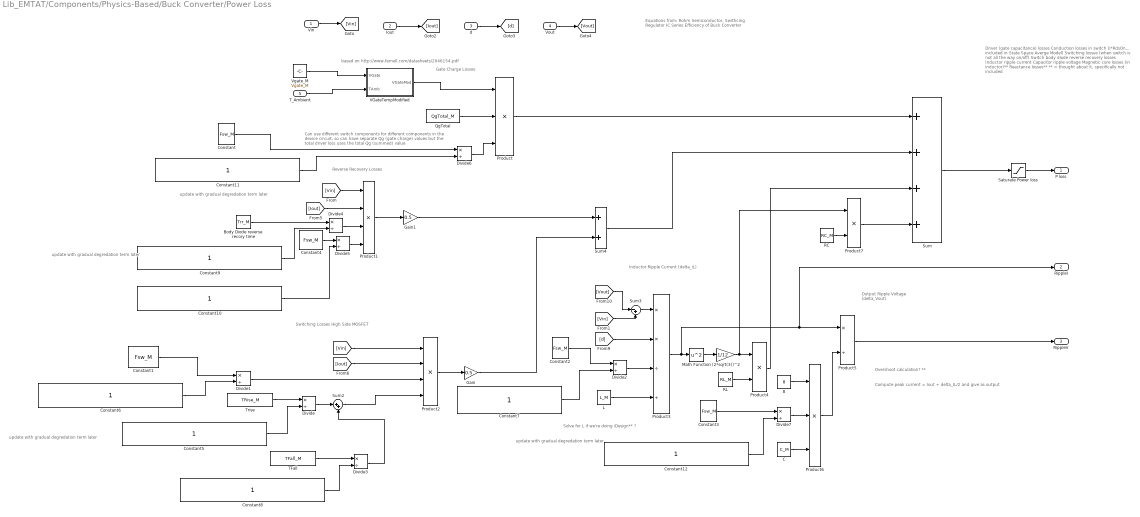
== system Lib_EMTAT/Components/Physics-Based/Buck Converter/Power Loss  ==
  note: Equations from:
      | Rohm Semiconductor, Swithcing Regulator IC Series
      | Efficiency of Buck Converter
  note: Compute peak current = Iout + delta_IL/2 and give as output
  note: Solve for L if we're doing iDesign** ?
  note: Gate Charge Losses
  note: Can use different switch components for different components in
      | the device circuit, so can have separate Qg (gate charge) values
      | but the total driver loss uses the total Qg (summed) value
  note: Driver (gate capacitance) losses
      | Conduction losses in switch (I*RdsOn... included in State Space Averge Model)
      | Switching losses (when switch is not all the way on/off)
      | Switch body diode reverse recovery losses
      | Inductor ripple current
      | Capacitor ripple voltage
      | Magnetic core losses (in inductor)**
      | Reactance losses**
      | ** = thought about it, specifically not included
  note: Switching Losses High Side MOSFET
  note: Reverse Recovery Losses
  note: Inductor Ripple Current
      | (delta_iL)
  note: Output Ripple Voltage
      | (delta_Vout)
  note: Overshoot calculation? **
  note: based on http://www.farnell.com/datasheets/2046154.pdf
  note: update with gradual degredation term later
  note: update with gradual degredation term later
  note: update with gradual degredation term later
  note: update with gradual degredation term later
  Vin : Inport
  Iout : Inport  Port=2
  d : Inport  Port=3
  Vout : Inport  Port=4
  "T_Ambient " : Inport  Port=5
  (2*sqrt(3))^2 : Gain  Gain=1/12
  8 : Constant  Value=8  VectorParams1D=off
  Body Diode reverse recory time : Constant  Value=Trr_M  VectorParams1D=off
  C : Constant  Value=C_M  VectorParams1D=off
  Constant{,1..4} (5 alike) : Constant  Value=Fsw_M
  Constant{5..12} (8 alike) : Constant
  Divide{,1..7} (8 alike) : Product  Inputs=*/
  Gain : Gain  Gain=0.5
  Gain1 : Gain  Gain=0.5
  L : Constant  Value=L_M  VectorParams1D=off
  Math Function : Math  Operator=square  SignedPower=on  SaturateOnIntegerOverflow=on
  Product : Product  Inputs=3
  Product1 : Product  Inputs=4
  Product2 : Product  Inputs=4
  Product3 : Product  Inputs=**//
  Product4 : Product
  Product5 : Product  Inputs=*/
  Product6 : Product  Inputs=3
  Product7 : Product
  QgTotal : Constant  Value=QgTotal_M  VectorParams1D=off
  RC : Constant  Value=RC_M  VectorParams1D=off
  RL : Constant  Value=RL_M  VectorParams1D=off
  Saturate Power loss : Saturate  UpperLimit=inf  LowerLimit=0
  Sum : Sum  Inputs=++++
  Sum2 : Sum  Inputs=|++
  Sum3 : Sum  Inputs=|-+
  Sum4 : Sum
  TFall : Constant  Value=TFall_M  VectorParams1D=off
  Trise : Constant  Value=TRise_M  VectorParams1D=off
  VGateTempModified : Subsystem
  Vgate_M : Constant  Value=Vgate_M
  " P loss" : Outport  VectorParamsAs1DForOutWhenUnconnected=off
  RippleI : Outport  Port=2  VectorParamsAs1DForOutWhenUnconnected=off
  RippleV : Outport  Port=3  VectorParamsAs1DForOutWhenUnconnected=off
  wires:
  Product7/1 -> Sum/4
  RC/1 -> Product7/2
  Product5/1 -> RippleV/1
  C/1 -> Product6/3
  8/1 -> Product6/1
  Product6/1 -> Product5/2
  Math Function/1 -> (2*sqrt(3))^2/1
  (2*sqrt(3))^2/1 -> Product4/1, Product7/1
  Product3/1 -> Math Function/1, RippleI/1, Product5/1
  RL/1 -> Product4/2
  Product4/1 -> Sum/3
  L/1 -> Product3/4
  Sum3/1 -> Product3/1
  Sum2/1 -> Product2/4
  Product/1 -> Sum/1
  Sum4/1 -> Sum/2
  QgTotal/1 -> Product/2
  Saturate Power loss/1 -> " P loss"/1
  Sum/1 -> Saturate Power loss/1
  Vin/1 -> [Vin]
  [Vin] -> Product2/1
  [Vin] -> Sum3/2
  Iout/1 -> [Iout]
  [Iout] -> Product2/2
  d/1 -> [d]
  [d] -> Product3/2
  Vout/1 -> [Vout]
  [Vout] -> Sum3/1
  Product2/1 -> Gain/1
  Gain/1 -> Sum4/2
  [Vin] -> Product1/1
  [Iout] -> Product1/2
  Product1/1 -> Gain1/1
  Gain1/1 -> Sum4/1
  Vgate_M/1 -> VGateTempModified/1("VGate ")
  "T_Ambient "/1 -> VGateTempModified/2(TAmb)
  VGateTempModified/1("VGateMod ") -> Product/1
  Divide/1 -> Sum2/1
  Trise/1 -> Divide/1
  Constant5/1 -> Divide/2
  Divide1/1 -> Product2/3
  Constant1/1 -> Divide1/1
  Constant6/1 -> Divide1/2
  Divide2/1 -> Product3/3
  Constant2/1 -> Divide2/1
  Constant7/1 -> Divide2/2
  Divide3/1 -> Sum2/2
  TFall/1 -> Divide3/1
  Constant8/1 -> Divide3/2
  Divide4/1 -> Product1/3
  Body Diode reverse recory time/1 -> Divide4/1
  Constant9/1 -> Divide4/2
  Divide5/1 -> Product1/4
  Constant4/1 -> Divide5/1
  Constant10/1 -> Divide5/2
  Divide6/1 -> Product/3
  Constant/1 -> Divide6/1
  Constant11/1 -> Divide6/2
  Divide7/1 -> Product6/2
  Constant3/1 -> Divide7/1
  Constant12/1 -> Divide7/2

== system Lib_EMTAT/Components/Physics-Based/Electrothermal_Battery_Model/Battery Core (w// Q) ==
  it_base : Inport
  I_Demand : Inport  Port=2
  Tavg : Inport  Port=3
  BatteryCore : Subsystem
  Constant1 : Constant  Value=SOC_Init_M
  Vout : Outport  VectorParamsAs1DForOutWhenUnconnected=off
  SOC : Outport  Port=2  VectorParamsAs1DForOutWhenUnconnected=off
  it : Outport  Port=3  VectorParamsAs1DForOutWhenUnconnected=off
  Heat_Generated : Outport  Port=4  VectorParamsAs1DForOutWhenUnconnected=off
  wires:
  I_Demand/1 -> BatteryCore/3("Battery Current (A) ")
  Constant1/1 -> BatteryCore/1("SOC Init (%) ")
  Tavg/1 -> BatteryCore/4("Tavg ")
  it_base/1 -> BatteryCore/2("it base (Ah) ")
  BatteryCore/2(it (Ah)) -> it/1
  BatteryCore/1(Battery Voltage (V)) -> Vout/1
  BatteryCore/3(SOC (%)) -> SOC/1
  BatteryCore/4(Heat_Generated) -> Heat_Generated/1

== system Lib_EMTAT/Components/Physics-Based/Electrothermal_Battery_Model/it_Dot = f(i) ==
  i : Inport
  Convert As/s to Ah/s : Gain  Gain=1/3600
  it_Dot : Outport  VectorParamsAs1DForOutWhenUnconnected=off
  wires:
  Convert As/s to Ah/s/1 -> it_Dot/1
  i/1 -> Convert As/s to Ah/s/1

== system Lib_EMTAT/Components/Physics-Based/Generator/Copper Losses ==
  Iq : Inport
  Id1 : Inport  Port=2
  Res_DF : Inport  Port=3
  Divide : Product  Inputs=/*
  Divide1 : Product  Inputs=*/
  Gain1 : Gain  Gain=R_s
  Gain2 : Gain  Gain=R_s
  Square1 : Math  Operator=square  SignedPower=on  SaturateOnIntegerOverflow=on
  Square2 : Math  Operator=square  SignedPower=on  SaturateOnIntegerOverflow=on
  Sum : Sum
  P_Cu : Outport  VectorParamsAs1DForOutWhenUnconnected=off
  wires:
  Sum/1 -> P_Cu/1
  Square1/1 -> Gain1/1
  Iq/1 -> Square1/1
  Divide1/1 -> Sum/2
  Divide/1 -> Sum/1
  Gain1/1 -> Divide1/1
  Res_DF/1 -> Divide1/2, Divide/1
  Gain2/1 -> Divide/2
  Id1/1 -> Square2/1
  Square2/1 -> Gain2/1

== system Lib_EMTAT/Components/Physics-Based/Generator/Field Weakening and d current  ==
  note: Needs: S_n,flux_m,L_s
  S : Inport
  Flux_DF : Inport  Port=2
  Constant : Constant  Value=flux_m
  Constant1 : Constant  Value=S_nom
  Divide : Product  Inputs=*/
  Gain : Gain  Gain=1/L_s
  Product : Product
  Product1 : Product
  Subtract : Sum  Inputs=+-
  Switch : Switch  Criteria=u2 > Threshold  Threshold=S_nom
  flux_s : Outport  VectorParamsAs1DForOutWhenUnconnected=off
  Id : Outport  Port=2  VectorParamsAs1DForOutWhenUnconnected=off
  wires:
  S/1 -> Divide/2, Switch/2
  Product/1 -> Switch/1
  Divide/1 -> Product/2
  Switch/1 -> Subtract/1, flux_s/1
  Subtract/1 -> Gain/1
  Gain/1 -> Id/1
  Product1/1 -> Switch/3, Product/1, Subtract/2
  Constant/1 -> Product1/1
  Flux_DF/1 -> Product1/2
  Constant1/1 -> Divide/1

== system Lib_EMTAT/Components/Physics-Based/Generator/I_rms (Actual) ==
  note: I_RMS (actual) = sqrt(Id^2 + Iq^2)
  iq : Inport
  id : Inport  Port=2
  Isign : Inport  Port=3
  Add : Sum
  Mult : Product  Inputs=**
  Square : Math  Operator=square  SaturateOnIntegerOverflow=on
  Square Root : Sqrt  SaturateOnIntegerOverflow=on
  Square1 : Math  Operator=square  SaturateOnIntegerOverflow=on
  to RMS : Gain  Gain=1/sqrt(3)
  Is : Outport
  wires:
  Add/1 -> Square Root/1
  Square/1 -> Add/1
  Mult/1 -> to RMS/1
  Isign/1 -> Mult/1
  to RMS/1 -> Is/1  "Is"
  Square Root/1 -> Mult/2
  iq/1 -> Square1/1
  Square1/1 -> Add/2
  id/1 -> Square/1

== system Lib_EMTAT/Components/Physics-Based/Generator/Iq ==
  Is : Inport
  Id : Inport  Port=2
  Add1 : Sum  Inputs=+-
  Square Root1 : Sqrt  SaturateOnIntegerOverflow=on
  Square2 : Math  Operator=square  SignedPower=on  SaturateOnIntegerOverflow=on
  Square3 : Math  Operator=square  SignedPower=on  SaturateOnIntegerOverflow=on
  Iq : Outport  VectorParamsAs1DForOutWhenUnconnected=off
  wires:
  Is/1 -> Square2/1
  Id/1 -> Square3/1
  Square2/1 -> Add1/1
  Square3/1 -> Add1/2
  Add1/1 -> Square Root1/1
  Square Root1/1 -> Iq/1

== system Lib_EMTAT/Components/Physics-Based/Generator/Iron Loss ==
  w_elec : Inport
  Constant : Constant  Value=S_nom*((2*pi)/60)*pp
  Divide : Product  Inputs=*/
  Gain : Gain  Gain=P_Fe_Nom
  P_Fe : Outport  VectorParamsAs1DForOutWhenUnconnected=off
  wires:
  Divide/1 -> Gain/1
  w_elec/1 -> Divide/1
  Gain/1 -> P_Fe/1
  Constant/1 -> Divide/2

== system Lib_EMTAT/Components/Physics-Based/Generator/Power Factor Calc ==
  Id : Inport
  Iq : Inport  Port=2
  Vd : Inport  Port=3
  Vq : Inport  Port=4
  P : Inport  Port=5
  Divide : Product  Inputs=*/
  Product : Product
  Product1 : Product
  Subtract : Sum  Inputs=+-
  Trigonometric Function : Trigonometry  Operator=atan
  Out1 : Outport  VectorParamsAs1DForOutWhenUnconnected=off
  wires:
  Trigonometric Function/1 -> Out1/1
  Divide/1 -> Trigonometric Function/1
  P/1 -> Divide/2
  Subtract/1 -> Divide/1
  Product/1 -> Subtract/1
  Product1/1 -> Subtract/2
  Iq/1 -> Product1/2
  Vd/1 -> Product1/1
  Id/1 -> Product/2
  Vq/1 -> Product/1

== system Lib_EMTAT/Components/Physics-Based/Generator/Torque Saturation Logic ==
  note: Needs: P_m_max, T_ref_max
  T_ref_in : Inport
  S : Inport  Port=2
  Abs : Abs
  Constant1 : Constant  Value=P_out_max
  Divide : Product  Inputs=*/
  Product : Product
  Sat (ft-lbs) : Saturate  UpperLimit=T_nom*1.3558  LowerLimit=-T_nom*1.3558
  Switch : Switch  Criteria=u2 > Threshold  Threshold=P_out_max
  T_ref_sat : Outport  VectorParamsAs1DForOutWhenUnconnected=off
  wires:
  T_ref_in/1 -> Sat (ft-lbs)/1, Product/1  "Nm"
  Constant1/1 -> Divide/1  "W"
  S/1 -> Product/2, Divide/2
  Abs/1 -> Switch/2  "W"
  Switch/1 -> T_ref_sat/1
  Sat (ft-lbs)/1 -> Switch/3  "Nm"
  Product/1 -> Abs/1  "W"
  Divide/1 -> Switch/1  "Nm"

== system Lib_EMTAT/Components/Physics-Based/Generator/Vdq ==
  Id : Inport
  w_elec : Inport  Port=2
  Iq : Inport  Port=3
  Res_DF : Inport  Port=4
  Flux_DF : Inport  Port=5
  Divide : Product  Inputs=*/
  Divide1 : Product  Inputs=/*
  Gain : Gain  Gain=R_s
  Gain1 : Gain  Gain=R_s
  Gain2 : Gain  Gain=L_s
  Gain3 : Gain  Gain=flux_m
  Product : Product
  Product1 : Product
  Product2 : Product
  Subtract : Sum  Inputs=+-
  Sum : Sum  Inputs=+++
  Vd : Outport  VectorParamsAs1DForOutWhenUnconnected=off
  Vq : Outport  Port=2  VectorParamsAs1DForOutWhenUnconnected=off
  wires:
  Id/1 -> Gain/1, Product1/1
  Iq/1 -> Gain1/1, Product/2
  w_elec/1 -> Gain2/1, Gain3/1
  Gain2/1 -> Product/1, Product1/2
  Product/1 -> Subtract/2
  Subtract/1 -> Vd/1
  Product1/1 -> Sum/1
  Sum/1 -> Vq/1
  Product2/1 -> Sum/3
  Gain3/1 -> Product2/1
  Divide/1 -> Sum/2
  Gain1/1 -> Divide/1
  Divide1/1 -> Subtract/1
  Flux_DF/1 -> Product2/2
  Gain/1 -> Divide1/2
  Res_DF/1 -> Divide/2, Divide1/1

== system Lib_EMTAT/Components/Physics-Based/Generator/Vs ==
  Vd : Inport
  Vq : Inport  Port=2
  Add : Sum
  Square : Math  Operator=square  SignedPower=on  SaturateOnIntegerOverflow=on
  Square Root : Sqrt  SaturateOnIntegerOverflow=on
  Square1 : Math  Operator=square  SignedPower=on  SaturateOnIntegerOverflow=on
  Vs : Outport  VectorParamsAs1DForOutWhenUnconnected=off
  wires:
  Square Root/1 -> Vs/1
  Add/1 -> Square Root/1
  Square/1 -> Add/2
  Square1/1 -> Add/1
  Vd/1 -> Square1/1
  Vq/1 -> Square/1

== system Lib_EMTAT/Components/Physics-Based/Inverter /Diode Conduction Losses ==
  note: the aDF must decrease u_D_M
  note: You need to read from graphs:
      |
      | -U_ce0
      | -Rc=dU_ce/dI_c (linear)
      | -U_D0
      | -R_D=dU_D/dI_D (linear)
  I_M : Inport
  PF : Inport  Port=2
  m : Inport  Port=3
  T : Inport  Port=4
  1-D Lookup Table r_D : Lookup_n-D  NumberOfTableDimensions=1  BreakpointsForDimension1=T_M  Table=R_D_M  InternalRulePriority=Speed  RndMeth=Simplest  InputSameDT=on
  1-D Lookup Table u_D0 : Lookup_n-D  NumberOfTableDimensions=1  BreakpointsForDimension1=T_M  Table=u_D_M  InternalRulePriority=Speed  RndMeth=Simplest  InputSameDT=on
  Constant : Constant  Value=1/(2*pi)
  Constant1 : Constant  Value=1/8
  Gain : Gain  Commented=on  Gain=u_D0
  Gain1 : Gain  Gain=1/8
  Gain2 : Gain  Commented=on  Gain=r_D
  Gain3 : Gain  Gain=1/(3*pi)
  Product{,1..4} (5 alike) : Product
  Square : Math  Operator=square  SignedPower=on  SaturateOnIntegerOverflow=on
  Sum : Sum  Inputs=+-
  Sum2 : Sum
  Sum3 : Sum  Inputs=-+
  P_CD : Outport  VectorParamsAs1DForOutWhenUnconnected=off
  wires:
  Product/1 -> Sum2/1
  Product2/1 -> Sum2/2
  Sum2/1 -> P_CD/1
  I_M/1 -> Product3/1  "I_M"
  Product3/1 -> Product/2, Square/1
  Constant/1 -> Sum/1
  PF/1 -> Product1/1
  m/1 -> Product1/2
  Gain1/1 -> Sum/2
  Product1/1 -> Gain3/1, Gain1/1
  Sum/1 -> Product/1
  Square/1 -> Product4/1
  Gain3/1 -> Sum3/1
  Product4/1 -> Product2/1
  Constant1/1 -> Sum3/2
  Sum3/1 -> Product2/2
  T/1 -> 1-D Lookup Table u_D0/1, 1-D Lookup Table r_D/1
  1-D Lookup Table u_D0/1 -> Product3/2
  1-D Lookup Table r_D/1 -> Product4/2

== system Lib_EMTAT/Components/Physics-Based/Inverter /Diode Switching Losses ==
  note: I_Drrpeak=2Qrr/trr
  note: Worst case - voltage across diode is supply voltage
  Input : Inport
  Constant1 : Constant  Value=f_sw
  Gain : Gain  Gain=.25*Q_rr
  Product2 : Product
  P_rec_D : Outport  VectorParamsAs1DForOutWhenUnconnected=off
  wires:
  Product2/1 -> P_rec_D/1
  Constant1/1 -> Product2/2  "I_M"
  Gain/1 -> Product2/1
  Input/1 -> Gain/1  "V_batt"

== system Lib_EMTAT/Components/Physics-Based/Inverter /IGBT Conduction Losses ==
  note: You need to read from graphs:
      |
      | -U_ce0
      | -Rc=dU_ce/dI_c (linear)
      | -U_D0
      | -R_D=dU_D/dI_D (linear)
  I_M : Inport
  PF : Inport  Port=2
  m : Inport  Port=3
  T : Inport  Port=4
  1-D Lookup Table r_c : Lookup_n-D  NumberOfTableDimensions=1  BreakpointsForDimension1=T_M  Table=R_c_M  InternalRulePriority=Speed  RndMeth=Simplest  InputSameDT=on
  1-D Lookup Table u_ce0 : Lookup_n-D  NumberOfTableDimensions=1  BreakpointsForDimension1=T_M  Table=u_ce0_M  InternalRulePriority=Speed  RndMeth=Simplest  InputSameDT=on
  Constant : Constant  Value=1/(2*pi)
  Constant1 : Constant  Value=1/8
  Gain : Gain  Commented=on  Gain=u_ce0
  Gain1 : Gain  Gain=1/8
  Gain2 : Gain  Commented=on  Gain=r_c
  Gain3 : Gain  Gain=1/(3*pi)
  Product{,1..4} (5 alike) : Product
  Square : Math  Operator=square  SignedPower=on  SaturateOnIntegerOverflow=on
  Sum : Sum
  Sum2 : Sum
  Sum3 : Sum
  P_CT : Outport  VectorParamsAs1DForOutWhenUnconnected=off
  wires:
  Product/1 -> Sum2/1
  Product2/1 -> Sum2/2
  Sum2/1 -> P_CT/1
  I_M/1 -> Product3/1  "I_M"
  Product3/1 -> Product/2, Square/1
  Constant/1 -> Sum/1
  PF/1 -> Product1/1
  m/1 -> Product1/2
  Gain1/1 -> Sum/2
  Product1/1 -> Gain3/1, Gain1/1
  Sum/1 -> Product/1
  Square/1 -> Product4/1
  Gain3/1 -> Sum3/1
  Product4/1 -> Product2/1
  Constant1/1 -> Sum3/2
  Sum3/1 -> Product2/2
  T/1 -> 1-D Lookup Table u_ce0/1, 1-D Lookup Table r_c/1
  1-D Lookup Table u_ce0/1 -> Product3/2
  1-D Lookup Table r_c/1 -> Product4/2

== system Lib_EMTAT/Components/Physics-Based/Inverter /IGBT Switching Losses ==
  note: the aDF must increase E1_M
  note: update with gradual degredation term later
  I_ce : Inport
  T : Inport  Port=2
  1-D Lookup Table E0 : Lookup_n-D  NumberOfTableDimensions=1  BreakpointsForDimension1=T_M  Table=E0_M  InternalRulePriority=Speed  RndMeth=Simplest  InputSameDT=on
  1-D Lookup Table E1 : Lookup_n-D  NumberOfTableDimensions=1  BreakpointsForDimension1=T_M  Table=E1_M  InternalRulePriority=Speed  RndMeth=Simplest  InputSameDT=on
  Add : Sum
  Constant : Constant  Value=f_sw_M
  Constant1 : Constant
  Divide : Product  Inputs=*/
  Product : Product
  Product1 : Product
  P_ST : Outport  VectorParamsAs1DForOutWhenUnconnected=off
  wires:
  Product/1 -> P_ST/1
  Add/1 -> Product/1
  I_ce/1 -> Product1/1
  1-D Lookup Table E0/1 -> Add/1
  Product1/1 -> Add/2
  T/1 -> 1-D Lookup Table E0/1, 1-D Lookup Table E1/1
  1-D Lookup Table E1/1 -> Product1/2
  Divide/1 -> Product/2
  Constant/1 -> Divide/1
  Constant1/1 -> Divide/2

== system Lib_EMTAT/Components/Physics-Based/Inverter /I_Ripple ==
  note: update with gradual degredation term later
  V_batt : Inport
  "V_M " : Inport  Port=2
  Constant : Constant  Value=L_s_M
  Constant1 : Constant
  Divide : Product  Inputs=*/
  Divide1 : Product  Inputs=*/
  Gain : Gain  Gain=sqrt(2)
  Gain1 : Gain  Gain=2
  Gain2 : Gain  Gain=f_sw_M
  Product : Product
  Product1 : Product
  Subtract : Sum  Inputs=+-
  Inport Value : Outport  VectorParamsAs1DForOutWhenUnconnected=off
  wires:
  "V_M "/1 -> Product/2, Gain/1
  Gain/1 -> Subtract/2
  V_batt/1 -> Subtract/1, Product1/1
  Subtract/1 -> Product/1
  Product/1 -> Divide/1
  Constant/1 -> Gain1/1
  Gain1/1 -> Product1/2
  Product1/1 -> Gain2/1
  Divide/1 -> Inport Value/1
  Divide1/1 -> Divide/2
  Gain2/1 -> Divide1/1
  Constant1/1 -> Divide1/2

== system Lib_EMTAT/Components/Physics-Based/Inverter /P_in_mot ==
  V_s : Inport
  I : Inport  Port=2
  PF : Inport  Port=3
  Gain : Gain  Gain=sqrt(3)
  Product : Product  Inputs=3
  P_in_mot : Outport  VectorParamsAs1DForOutWhenUnconnected=off
  wires:
  I/1 -> Product/2
  PF/1 -> Product/3
  V_s/1 -> Product/1
  Gain/1 -> P_in_mot/1
  Product/1 -> Gain/1

== system Lib_EMTAT/Components/Physics-Based/Inverter /mVal ==
  V_s : Inport
  V_batt : Inport  Port=2
  Divide : Product  Inputs=*/
  Gain : Gain  Gain=sqrt(2)
  m : Outport  VectorParamsAs1DForOutWhenUnconnected=off
  V_batt_pass : Outport  Port=2  VectorParamsAs1DForOutWhenUnconnected=off
  wires:
  Divide/1 -> m/1
  V_s/1 -> Gain/1
  Gain/1 -> Divide/1
  V_batt/1 -> V_batt_pass/1, Divide/2

== system Lib_EMTAT/Components/Physics-Based/Motor /Copper Losses ==
  Id : Inport
  Iq : Inport  Port=2
  Flux_DF : Inport  Port=3
  Res_DF : Inport  Port=4
  Divide : Product  Inputs=*/
  Divide1 : Product  Inputs=/*
  Gain : Gain  Gain=R_s
  Gain1 : Gain  Gain=R_s
  Square : Math  Operator=square  SignedPower=on  SaturateOnIntegerOverflow=on
  Square1 : Math  Operator=square  SignedPower=on  SaturateOnIntegerOverflow=on
  Sum : Sum
  P_Cu : Outport  VectorParamsAs1DForOutWhenUnconnected=off
  wires:
  Iq/1 -> Square1/1
  Id/1 -> Square/1
  Square/1 -> Gain/1
  Square1/1 -> Gain1/1
  Sum/1 -> P_Cu/1
  Gain1/1 -> Divide/1
  Flux_DF/1 -> Divide/2
  Gain/1 -> Divide1/2
  Divide1/1 -> Sum/1
  Divide/1 -> Sum/2
  Res_DF/1 -> Divide1/1

== system Lib_EMTAT/Components/Physics-Based/Motor /Field Weakening and d current  ==
  note: Needs: S_n,flux_m,L_s
  S : Inport
  Flux_DF : Inport  Port=2
  Constant : Constant  Value=flux_m
  Constant1 : Constant  Value=S_nom
  Divide : Product  Inputs=*/
  Gain : Gain  Gain=1/L_s
  Product : Product
  Product1 : Product
  Subtract : Sum  Inputs=+-
  Switch : Switch  Criteria=u2 > Threshold  Threshold=S_nom
  flux_s : Outport  VectorParamsAs1DForOutWhenUnconnected=off
  id : Outport  Port=2  VectorParamsAs1DForOutWhenUnconnected=off
  wires:
  S/1 -> Divide/2, Switch/2
  Product/1 -> Switch/1
  Divide/1 -> Product/2
  Switch/1 -> Subtract/1, flux_s/1
  Subtract/1 -> Gain/1
  Gain/1 -> id/1
  Constant/1 -> Product1/1
  Product1/1 -> Subtract/2, Product/1, Switch/3
  Flux_DF/1 -> Product1/2
  Constant1/1 -> Divide/1

== system Lib_EMTAT/Components/Physics-Based/Motor /Iron Loss ==
  w_elec : Inport
  Constant : Constant  Value=S_nom*((2*pi)/60)*pp
  Divide : Product  Inputs=*/
  Gain : Gain  Gain=P_Fe_Nom
  P_Fe : Outport  VectorParamsAs1DForOutWhenUnconnected=off
  wires:
  w_elec/1 -> Divide/1
  Divide/1 -> Gain/1
  Gain/1 -> P_Fe/1
  Constant/1 -> Divide/2

== system Lib_EMTAT/Components/Physics-Based/Motor /Is ==
  Id : Inport
  Iq : Inport  Port=2
  Add : Sum
  Square : Math  Operator=square  SignedPower=on  SaturateOnIntegerOverflow=on
  Square Root : Sqrt  SaturateOnIntegerOverflow=on
  Square1 : Math  Operator=square  SignedPower=on  SaturateOnIntegerOverflow=on
  Is : Outport  VectorParamsAs1DForOutWhenUnconnected=off
  wires:
  Iq/1 -> Square/1
  Id/1 -> Square1/1
  Square1/1 -> Add/1
  Square/1 -> Add/2
  Add/1 -> Square Root/1
  Square Root/1 -> Is/1

== system Lib_EMTAT/Components/Physics-Based/Motor /Power Factor Calc  ==
  Id : Inport
  Iq : Inport  Port=2
  Vd : Inport  Port=3
  Vq : Inport  Port=4
  P : Inport  Port=5
  Display : Display
  Divide : Product  Inputs=*/
  Product : Product
  Product1 : Product
  Subtract : Sum  Inputs=+-
  Trigonometric Function : Trigonometry  Operator=atan
  Out1 : Outport  VectorParamsAs1DForOutWhenUnconnected=off
  wires:
  Vq/1 -> Product/1
  Id/1 -> Product/2
  Vd/1 -> Product1/1
  Iq/1 -> Product1/2
  Product1/1 -> Subtract/2
  Product/1 -> Subtract/1
  Subtract/1 -> Divide/1
  P/1 -> Divide/2, Display/1
  Divide/1 -> Trigonometric Function/1
  Trigonometric Function/1 -> Out1/1
